simulink model "mux_axi"  (R2019b)
settings: Solver=FixedStepDiscrete  StartTime=0.0  StopTime=1e-7  RelTol=1e-3
undefined symbols (not defined in the file): t_clk
libraries: hdlsllib x9, simulink x2
settings Model: DataTypeOverride=Off  Creator=ga92wum  LastModifiedBy=ga92wum
settings DataIOCC: LimitDataPoints=on  SaveOutput=off  SaveTime=off
settings OptimizationCC: BlockReduction=off  ConditionallyExecuteInputs=off  DefaultParameterBehavior=Inlined  LifeSpan=inf
settings DebuggingCC: AlgebraicLoopMsg=error  SingleTaskRateTransMsg=error  AllowSymbolicDim=off  StrictBusMsg=ErrorOnBusTreatedAsVector  SFUnexpectedBacktrackingDiag=warning  SFNoUnconditionalDefaultTransitionDiag=warning  SFExecutionAtInitializationDiag=none  ArithmeticOperatorsInVariantConditions=warning
settings HardwareCC: ProdBitPerPointer=32  ProdBitPerSizeT=32  ProdBitPerPtrDiffT=32  ProdLargestAtomicFloat=None  ProdIntDivRoundTo=Undefined  ProdEndianess=Unspecified  ProdWordSize=32  ProdHWDeviceType=ASIC/FPGA->ASIC/FPGA  ProdEqTarget=off
settings SFSimCC: SimUseLocalCustomCode=off  CustomCodeUndefinedFunction=UseInterfaceOnly
settings RTWCC: RTWUseLocalCustomCode=off
settings CodeAppCC: StateflowObjectComments=on
settings GRTTargetCC: TargetLangStandard=C89/C90 (ANSI)  GeneratePreprocessorConditionals=Disable all
settings ConfigComp: CovScope=ReferencedModels  CovMetricSettings=dw  CovHtmlReporting=on  CovSaveCumulativeToWorkspaceVar=on  CovSaveSingleToWorkspaceVar=on  CovExternalEMLEnable=off  CovSFcnEnable=off

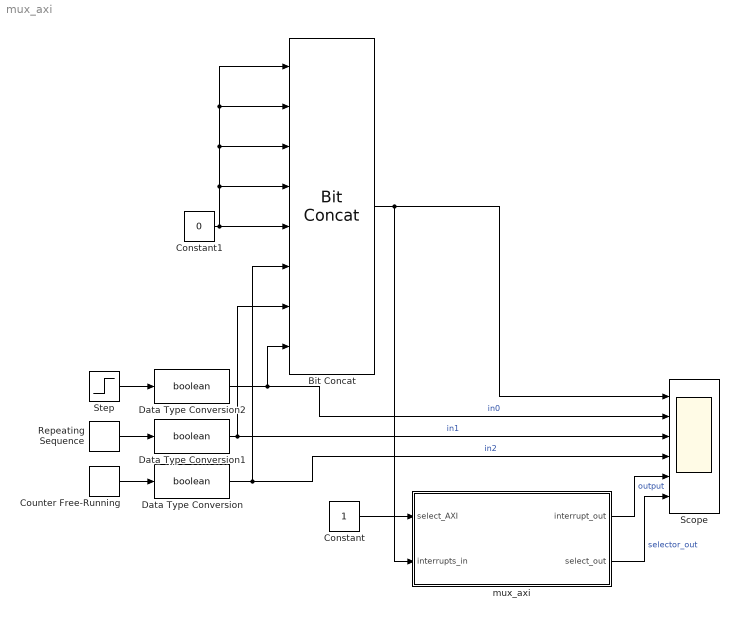
== system mux_axi ==
  Bit Concat : hdlsllib/Logic and Bit Operations/Bit Concat  numInputs=8
      settings: SourceProductName=Simulink
  Constant : Constant  OutDataTypeStr=uint32  SampleTime=-1
  Constant1 : Constant  Value=0  OutDataTypeStr=boolean  SampleTime=-1
  Counter Free-Running : simulink/Sources/Counter Free-Running  NumBits=1  tsamp=t_clk
  Data Type Conversion : DataTypeConversion  OutDataTypeStr=boolean
  Data Type Conversion1 : DataTypeConversion  OutDataTypeStr=boolean
  Data Type Conversion2 : DataTypeConversion  OutDataTypeStr=boolean
  Repeating Sequence : simulink/Sources/Repeating Sequence  rep_seq_t=[0 4*t_clk]  rep_seq_y=[0 1]
  Scope : Scope  NumInputPorts=6
  Step : Step  Time=5*t_clk  SampleTime=t_clk
  mux_axi : Subsystem  TreatAsAtomicUnit=on
  wires:
  Data Type Conversion/1 -> Bit Concat/6, Scope/4  "in2"
  Repeating Sequence/1 -> Data Type Conversion1/1
  mux_axi/1(interrupt_out) -> Scope/5  "output"
  Step/1 -> Data Type Conversion2/1
  Constant/1 -> mux_axi/1(select_AXI)
  Counter Free-Running/1 -> Data Type Conversion/1
  mux_axi/2(select_out) -> Scope/6  "selector_out"
  Data Type Conversion2/1 -> Bit Concat/8, Scope/2  "in0"
  Data Type Conversion1/1 -> Bit Concat/7, Scope/3  "in1"
  Bit Concat/1 -> Scope/1, mux_axi/2(interrupts_in)
  Constant1/1 -> Bit Concat/2, Bit Concat/1, Bit Concat/3, Bit Concat/4, Bit Concat/5

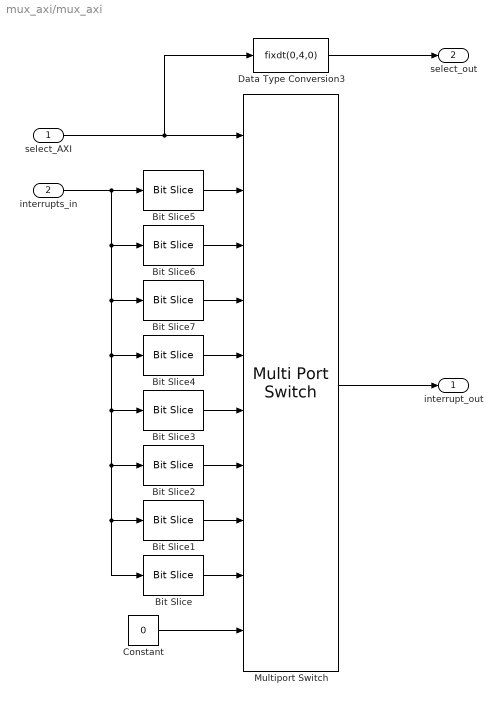
== system mux_axi/mux_axi ==
  select_AXI : Inport
  interrupts_in : Inport  Port=2  OutDataTypeStr=uint8
  Bit Slice : hdlsllib/Logic and Bit Operations/Bit Slice  lidx=7  ridx=7
      settings: SourceProductName=Simulink  SourceProductBaseCode=SL
  Bit Slice1 : hdlsllib/Logic and Bit Operations/Bit Slice  lidx=6  ridx=6
      settings: SourceProductName=Simulink  SourceProductBaseCode=SL
  Bit Slice2 : hdlsllib/Logic and Bit Operations/Bit Slice  lidx=5  ridx=5
      settings: SourceProductName=Simulink  SourceProductBaseCode=SL
  Bit Slice3 : hdlsllib/Logic and Bit Operations/Bit Slice  lidx=4  ridx=4
      settings: SourceProductName=Simulink  SourceProductBaseCode=SL
  Bit Slice4 : hdlsllib/Logic and Bit Operations/Bit Slice  lidx=3  ridx=3
      settings: SourceProductName=Simulink  SourceProductBaseCode=SL
  Bit Slice5 : hdlsllib/Logic and Bit Operations/Bit Slice  lidx=0  ridx=0
      settings: SourceProductName=Simulink  SourceProductBaseCode=SL
  Bit Slice6 : hdlsllib/Logic and Bit Operations/Bit Slice  lidx=1  ridx=1
      settings: SourceProductName=Simulink  SourceProductBaseCode=SL
  Bit Slice7 : hdlsllib/Logic and Bit Operations/Bit Slice  lidx=2  ridx=2
      settings: SourceProductName=Simulink  SourceProductBaseCode=SL
  Constant : Constant  Value=0  OutDataTypeStr=boolean  SampleTime=t_clk
  Data Type Conversion3 : DataTypeConversion  OutDataTypeStr=fixdt(0,4,0)
  Multiport Switch : MultiPortSwitch  DataPortOrder=Zero-based contiguous  Inputs=8  DataPortForDefault=Additional data port  zeroidx=on
  interrupt_out : Outport  OutDataTypeStr=boolean  VectorParamsAs1DForOutWhenUnconnected=off
  select_out : Outport  Port=2  VectorParamsAs1DForOutWhenUnconnected=off
  wires:
  Multiport Switch/1 -> interrupt_out/1
  Bit Slice3/1 -> Multiport Switch/6
  Bit Slice2/1 -> Multiport Switch/7
  Bit Slice4/1 -> Multiport Switch/5
  Bit Slice7/1 -> Multiport Switch/4
  Bit Slice6/1 -> Multiport Switch/3
  Bit Slice5/1 -> Multiport Switch/2
  select_AXI/1 -> Data Type Conversion3/1, Multiport Switch/1
  interrupts_in/1 -> Bit Slice/1, Bit Slice1/1, Bit Slice2/1, Bit Slice3/1, Bit Slice4/1, Bit Slice7/1, Bit Slice6/1, Bit Slice5/1
  Bit Slice/1 -> Multiport Switch/9
  Constant/1 -> Multiport Switch/10
  Bit Slice1/1 -> Multiport Switch/8
  Data Type Conversion3/1 -> select_out/1
